simulink model "celsiusConverter_NicholasSeecharan"  (R2025b)
settings: Solver=VariableStepAuto  StartTime=0.0  StopTime=10.0  RelTol=1e-3

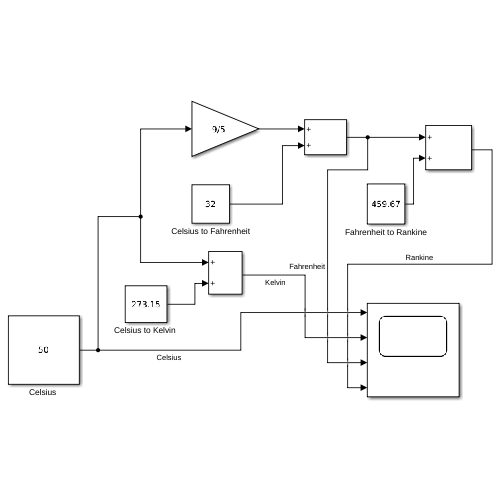
[thumbnail: Simulink's stored preview of the top-level diagram]
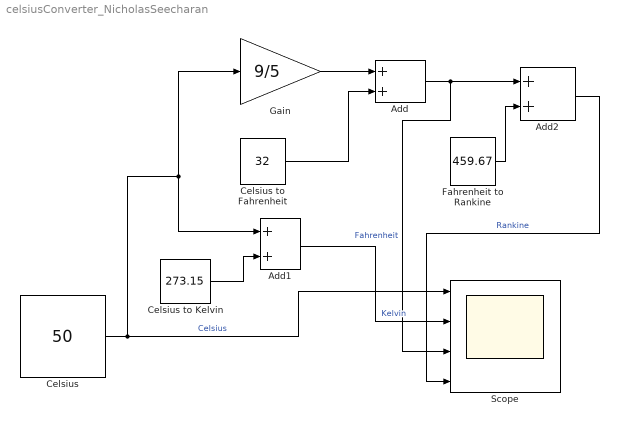
== system celsiusConverter_NicholasSeecharan ==
  Add : Sum
  Add1 : Sum
  Add2 : Sum
  "Celsius " : Constant  Value=50
  Celsius to Fahrenheit : Constant  Value=32
  "Celsius to Kelvin " : Constant  Value=273.15
  Fahrenheit to Rankine : Constant  Value=459.67
  Gain : Gain  Gain=9/5
  Scope : Scope  NumInputPorts=4
      settings: SampleTime=10  ActiveDisplayYMinimum=0  ActiveDisplayYMaximum=600
  wires:
  "Celsius "/1 -> Scope/1, Gain/1, Add1/1  "Celsius"
  Gain/1 -> Add/1
  Celsius to Fahrenheit/1 -> Add/2
  "Celsius to Kelvin "/1 -> Add1/2
  Add/1 -> Scope/3, Add2/1  "Fahrenheit"
  Fahrenheit to Rankine/1 -> Add2/2
  Add2/1 -> Scope/4  "Rankine"
  Add1/1 -> Scope/2  "Kelvin"
